simulink model "RC_RC_bipolar"  (R2013a)
settings: Solver=ode3  SolverMode=SingleTasking  StartTime=0.0  StopTime=10e-3  FixedStep=FS/50  MaxStep=1e-4  RelTol=1e-3
InitFcn:
  | %%%%%%  set scope time range
  | T_STOP=str2num(get_param(gcs,'StopTime'));
  | if numel(T_STOP) > 1
  |    T_STOP=T_STOP(2);
  | else
  |    T_STOP=T_STOP(1);
  | end
  | T_STOP=num2str(T_STOP);
  | 
  | %%%%%%  set scope time range in system @init_callback_fct
  | T_STOP=num2str(str2num(get_param(gcs,'StopTime')));
  | 
  | childs = allchild(0);
  | sol=strfind(upper(get(allchild(0),'Tag')),'VIEWER_PARAMETERS');
  | 
  | if iscell(sol)
  |    ind=find(~cellfun(@isempty, strfind(upper(get(allchild(0),'Tag')),'VIEWER_PARAMETERS')));
  | else
  |    ind=sol;
  | end
  | %ind=find(~cellfun(@isempty, {strfind(upper(get(allchild(0),'Tag')),'VIEWER_PARAMETERS'),[]}))
  | if ~isempty(ind)
  |    for k=1:length(childs(ind))
  |       set_param(getfield(get(childs(ind(k)),'UserData'),'block'),'TimeRange',T_STOP);
  |       get_param(getfield(get(childs(ind(k)),'UserData'),'block'),'TimeRange');
  | %    set_param(getfield(get(childs(ind),'UserData'),'block'),'TimeRange',T_STOP);
  | %    get_param(getfield(get(childs(ind),'UserData'),'block'),'TimeRange');
  |    end
  | else
  |     warning(sprintf('VIEWER_PARAMETERS object not found\nOpen the config dialog by hand for the first sim start'))
  | end
undefined symbols (not defined in the file or in its folder): Aw, FS, Lc, Rc, Rsh, T1
libraries: simulink x1
settings Model: BufferReuse=off  Creator=mainster  LastModifiedBy=mainster
settings SolverCC: AutoInsertRateTranBlk=on
settings OptimizationCC: InlineParams=on  BufferReuse=off
settings DebuggingCC: InitInArrayFormatMsg=none
settings HardwareCC: ProdLargestAtomicInteger=Long  ProdLargestAtomicFloat=Double  ProdEndianess=LittleEndian  ProdHWDeviceType=ARM Compatible->ARM Cortex

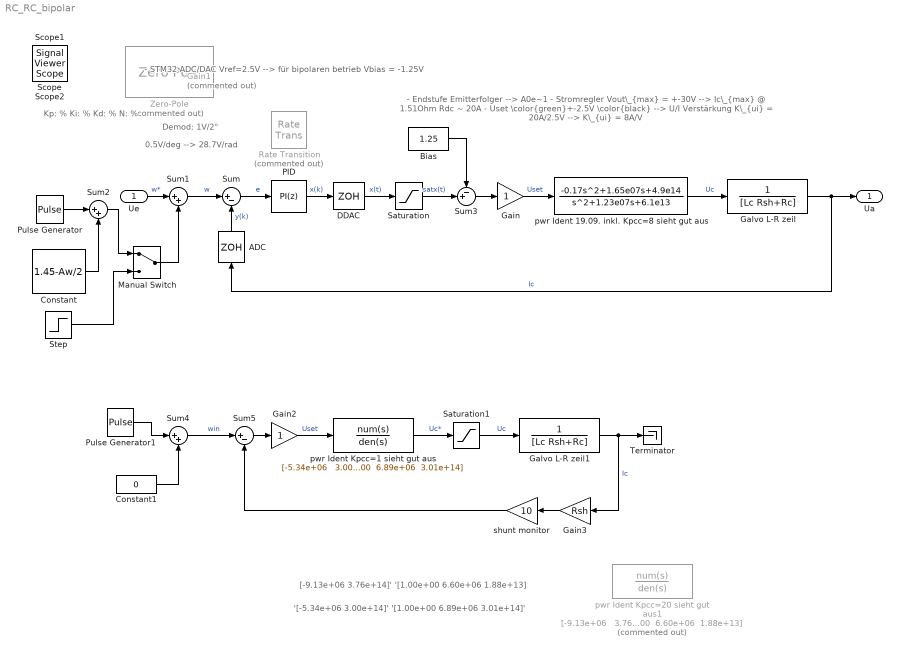
== system RC_RC_bipolar ==
  note: '[-5.34e+06 3.00e+14]' '[1.00e+00 6.89e+06 3.01e+14]'
  note: [-9.13e+06 3.76e+14]' '[1.00e+00 6.60e+06 1.88e+13]
  note: - Endstufe Emitterfolger --> A0e~1
      | - Stromregler Vout\_{max} = +-30V
      |       --> Ic\_{max} @ 1.51Ohm Rdc ~ 20A
      | - Uset \color{green}+-2.5V \color{black}
      |       --> U/I Verstärkung K\_{ui} = 20A/2.5V
      |       --> K\_{ui} = 8A/V
  note: - STM32 ADC/DAC Vref=2.5V
      | --> für bipolaren betrieb Vbias = -1.25V
  note: Kp: % Ki: % Kd: % N: %
  note: 0.5V/deg --> 28.7V/rad
  note: Demod:
      | 1V/2°
  Ue : Inport  SampleTime=FS
  ADC : ZeroOrderHold  SampleTime=FS
  Bias : Constant  Value=1.25  SampleTime=FS
  Constant : Constant  Value=1.45-Aw/2  SampleTime=FS
  Constant1 : Constant  Value=0  SampleTime=FS
  DDAC : ZeroOrderHold  SampleTime=FS
      settings: AttributesFormatString=%<SampleTime>
  Gain : Gain
  Gain1 : Gain  Commented=on  Gain=2
  Gain2 : Gain
  Gain3 : Gain  Gain=Rsh
  Galvo L-R zeil : TransferFcn  Numerator=1  Denominator=[Lc Rsh+Rc]
  Galvo L-R zeil1 : TransferFcn  Numerator=1  Denominator=[Lc Rsh+Rc]
  Manual Switch : ManualSwitch  SampleTime=FS
  "PID " : simulink/Continuous/PID Controller  Controller=PI  TimeDomain=Discrete-time  SampleTime=FS  IntegratorMethod=Forward Euler  FilterMethod=Forward Euler  Form=Parallel  P=1.84546966370507  I=3745.38790742202  D=9.0248898483108e-05  N=10930.7783722874  InitialConditionSource=internal  InitialConditionForIntegrator=0  InitialConditionForFilter=0  ExternalReset=none  LimitOutput=on  UpperSaturationLimit=1.25  LowerSaturationLimit=-1.25  LinearizeAsGain=on  AntiWindupMode=clamping  Kb=1  TrackingMode=off  Kt=1  PParamMin=[]  PParamMax=[]  IParamMin=[]  IParamMax=[]  DParamMin=[]  DParamMax=[]  NParamMin=[]  NParamMax=[]  KbParamMin=[]  KbParamMax=[]  KtParamMin=[]  KtParamMax=[]  POutMin=[]  POutMax=[]  IOutMin=[]  IOutMax=[]  DOutMin=[]  DOutMax=[]  NOutMin=[]  NOutMax=[]  KbOutMin=[]  KbOutMax=[]  KtOutMin=[]  KtOutMax=[]  IntegratorOutMin=[]  IntegratorOutMax=[]  FilterOutMin=[]  FilterOutMax=[]  SumOutMin=[]  SumOutMax=[]  SumI1OutMin=[]  SumI1OutMax=[]  SumI2OutMin=[]  SumI2OutMax=[]  SumI3OutMin=[]  SumI3OutMax=[]  SumDOutMin=[]  SumDOutMax=[]  SaturationOutMin=[]  SaturationOutMax=[]  IntegratorContinuousStateAttributes=''  IntegratorStateMustResolveToSignalObject=off  IntegratorRTWStateStorageClass=Auto  FilterContinuousStateAttributes=''  FilterStateMustResolveToSignalObject=off  FilterRTWStateStorageClass=Auto
  Pulse Generator : DiscretePulseGenerator  PulseType=Time based  Amplitude=Aw  Period=1/200  PulseWidth=50  PhaseDelay=0.5e-3  SampleTime=FS
  Pulse Generator1 : DiscretePulseGenerator  PulseType=Time based  Period=5e-3  PulseWidth=50  SampleTime=FS
  Rate Transition : RateTransition  Commented=on  OutPortSampleTime=FS
  Saturation : Saturate  UpperLimit=1.25  LowerLimit=-1.25
      settings: AttributesFormatString=Up_lim=%<UpperLimit>\nLo_lim=%<LowerLimit>
  Saturation1 : Saturate  UpperLimit=30  LowerLimit=-30
      settings: AttributesFormatString=Up_lim=%<UpperLimit>\nLo_lim=%<LowerLimit>
  Step : Step  Time=1e-3  SampleTime=FS
      settings: AttributesFormatString=Time:%<Time>\nAmp:%<After>
  Sum : Sum  Inputs=|+-  SampleTime=FS
  Sum1 : Sum  Inputs=|++  SampleTime=FS
  Sum2 : Sum  Inputs=|++  SampleTime=FS
  Sum3 : Sum  Inputs=-+|  SampleTime=FS
  Sum4 : Sum  Inputs=|++  SampleTime=FS
  Sum5 : Sum  Inputs=|+-  SampleTime=FS
  Terminator : Terminator
  Zero-Pole : ZeroPole  Commented=on  Zeros=[]  Poles=[-1/T1 -1/T1]  Gain=(1/T1)^2
  pwr Ident 19.09. inkl. Kpcc=8 sieht gut aus : TransferFcn  Numerator=|  Denominator="[1  1.23e07  6.1e13]"
      | [-0.17  1.65e07  4.9e14
      | ]
  pwr Ident Kpcc=1 sieht gut aus : TransferFcn  Numerator="[-5.34e+06   3.00e+14]"  Denominator="[1.00e+00  6.89e+06  3.01e+14]"
  pwr Ident Kpcc=20 sieht gut aus1 : TransferFcn  Commented=on  Numerator="[-9.13e+06   3.76e+14]"  Denominator="[1.00e+00  6.60e+06  1.88e+13]"
  shunt monitor : Gain  Gain=10
  Ua : Outport  SampleTime=FS
  Scope : SignalViewerScope  IOType=viewer  NumInputPorts=3  LegendLocations=|  RefreshTime=0.035000
      | 0.83845     0.92277     0.12384    0.036994
      | 0.83845     0.62331     0.12384    0.020768
      | 0.81611     0.30763     0.14618    0.020768
      settings: ShowLegends=on  TimeRange=0.01  YMin=-5~-5~-5  YMax=5~5~5
  Scope1 : SignalViewerScope  IOType=viewer  LegendLocations="0.80742     0.84238     0.15391    0.089755"  RefreshTime=0.035000
      settings: ShowLegends=on  TimeRange=0.01
  Scope2 : SignalViewerScope  IOType=viewer  NumInputPorts=3  LegendLocations=|  RefreshTime=0.035000
      | 0.80895     0.91959     0.13628    0.038514
      | 0.83054     0.62189     0.11545    0.021622
      | 0.83054     0.30622     0.11545    0.021622
      settings: ShowLegends=on  TimeRange=0.005  YMin=-1.5~-2~-0.4  YMax=1.5~2~0.4  SaveName=ScopeData2
  wires:
  Sum/1 -> "PID "/1  "e"
  Sum1/1 -> Sum/1  "w"
  Ue/1 -> Sum1/1  "w*"
  Galvo L-R zeil/1 -> Ua/1, ADC/1  "Ic"
  "PID "/1 -> DDAC/1  "x(k)"
  ADC/1 -> Sum/2  "y(k)"
  Step/1 -> Manual Switch/2
  Manual Switch/1 -> Sum1/2
  Sum2/1 -> Manual Switch/1
  Pulse Generator/1 -> Sum2/1
  Constant/1 -> Sum2/2
  Gain/1 -> pwr Ident 19.09. inkl. Kpcc=8 sieht gut aus/1  "Uset"
  pwr Ident 19.09. inkl. Kpcc=8 sieht gut aus/1 -> Galvo L-R zeil/1  "Uc"
  Saturation/1 -> Sum3/2  "satx(t)"
  Bias/1 -> Sum3/1
  Sum3/1 -> Gain/1
  DDAC/1 -> Saturation/1  "x(t)"
  Gain2/1 -> pwr Ident Kpcc=1 sieht gut aus/1  "Uset"
  pwr Ident Kpcc=1 sieht gut aus/1 -> Saturation1/1  "Uc*"
  Galvo L-R zeil1/1 -> Gain3/1, Terminator/1  "Ic"
  Pulse Generator1/1 -> Sum4/1
  Constant1/1 -> Sum4/2
  Sum4/1 -> Sum5/1  "win"
  Sum5/1 -> Gain2/1
  Saturation1/1 -> Galvo L-R zeil1/1  "Uc"
  Gain3/1 -> shunt monitor/1
  shunt monitor/1 -> Sum5/2
